simulink model "closed_loop_sim_est"  (R2024a)
settings: Solver=ode45  StartTime=0.0  StopTime=10  MaxStep=0.01  RelTol=1e-6
undefined symbols (not defined in the file): K_lat, K_long, X0
settings Model: Creator=mkaarthi  LastModifiedBy=mkaarthi

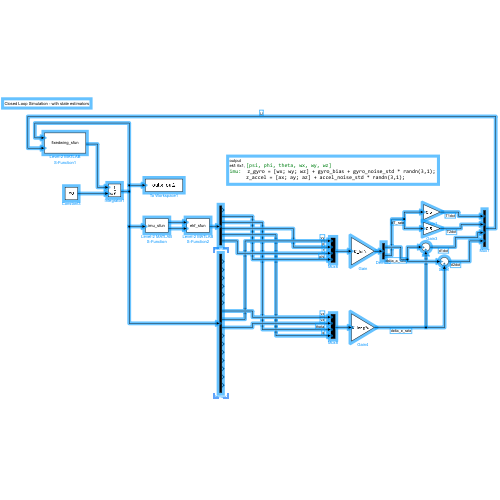
[thumbnail: Simulink's stored preview of the top-level diagram]
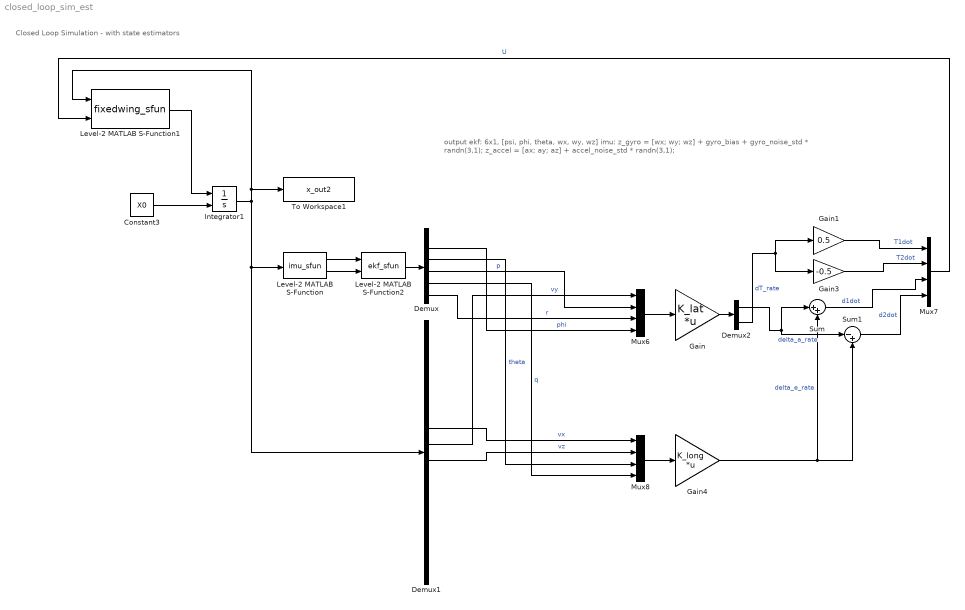
== system closed_loop_sim_est ==
  note: output
      | ekf: 6x1, [psi, phi, theta, wx, wy, wz]
      | imu: z_gyro = [wx; wy; wz] + gyro_bias + gyro_noise_std * randn(3,1);
      | z_accel = [ax; ay; az] + accel_noise_std * randn(3,1);
  note: Closed Loop Simulation - with state estimators
  Constant3 : Constant  Value=X0
  Demux : Demux  Outputs=6
  Demux1 : Demux  Outputs=16
  Demux2 : Demux  Outputs=2
  Gain : Gain  Gain=K_lat  Multiplication=Matrix(K*u)
  Gain1 : Gain  Gain=0.5
  Gain3 : Gain  Gain=-0.5
  Gain4 : Gain  Gain=K_long  Multiplication=Matrix(K*u)
  Integrator1 : Integrator  InitialConditionSource=external
  Level-2 MATLAB S-Function : M-S-Function  FunctionName=imu_sfun
  Level-2 MATLAB S-Function1 : M-S-Function  FunctionName=fixedwing_sfun
  Level-2 MATLAB S-Function2 : M-S-Function  FunctionName=ekf_sfun
  Mux6 : Mux
  Mux7 : Mux
  Mux8 : Mux
  Sum : Sum  Inputs=|++
  Sum1 : Sum  Inputs=|-+
  To Workspace1 : ToWorkspace  VariableName=x_out2  SampleTime=-1
  wires:
  Level-2 MATLAB S-Function1/1 -> Integrator1/1
  Demux2/1 -> Sum1/1, Sum/1  "delta_a_rate"
  Demux1/9 -> Mux8/2  "vz"
  Sum1/1 -> Mux7/4  "d2dot"
  Gain3/1 -> Mux7/2  "T2dot"
  Demux2/2 -> Gain3/1, Gain1/1  "dT_rate"
  Gain4/1 -> Sum/2, Sum1/2  "delta_e_rate"
  Mux6/1 -> Gain/1
  Gain1/1 -> Mux7/1  "T1dot"
  Demux1/8 -> Mux6/1  "vy"
  Integrator1/1 -> Demux1/1, Level-2 MATLAB S-Function/1, To Workspace1/1, Level-2 MATLAB S-Function1/1
  Constant3/1 -> Integrator1/2
  Sum/1 -> Mux7/3  "d1dot"
  Mux7/1 -> Level-2 MATLAB S-Function1/2  "U"
  Mux8/1 -> Gain4/1
  Demux1/7 -> Mux8/1  "vx"
  Gain/1 -> Demux2/1
  Level-2 MATLAB S-Function/1 -> Level-2 MATLAB S-Function2/1
  Level-2 MATLAB S-Function/2 -> Level-2 MATLAB S-Function2/2
  Level-2 MATLAB S-Function2/1 -> Demux/1
  Demux/2 -> Mux6/4  "phi"
  Demux/3 -> Mux8/3  "theta"
  Demux/4 -> Mux6/2  "p"
  Demux/5 -> Mux8/4  "q"
  Demux/6 -> Mux6/3  "r"
